simulink model "test"  (R2024a)
settings: Solver=ode1  StartTime=0.0  StopTime=4  FixedStep=0.0001  RelTol=1e-3  EnableMultiTasking=on
values from neighbouring files (symbols this model uses):
  kp = x(1)    [flc_error_ffunc.m]    (also in pi_regulator_ga_pso.m = wartosci_obliczone(1))
  ti = x(2)    [flc_error_ffunc.m]    (also in pi_regulator_ga_pso.m = wartosci_obliczone(2))
settings Model: Creator=poluser  LastModifiedBy=Hiver
settings DataIOCC: SaveOutput=off  SignalLogging=off  DSMLogging=off  SaveTime=off  ReturnWorkspaceOutputs=off
settings OptimizationCC: ReuseModelBlockBuffer=off
settings RTWCC: GPUComputeCapability=3.5

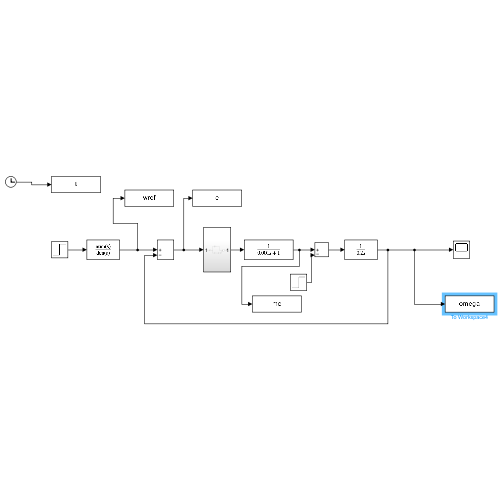
[thumbnail: Simulink's stored preview of the top-level diagram]
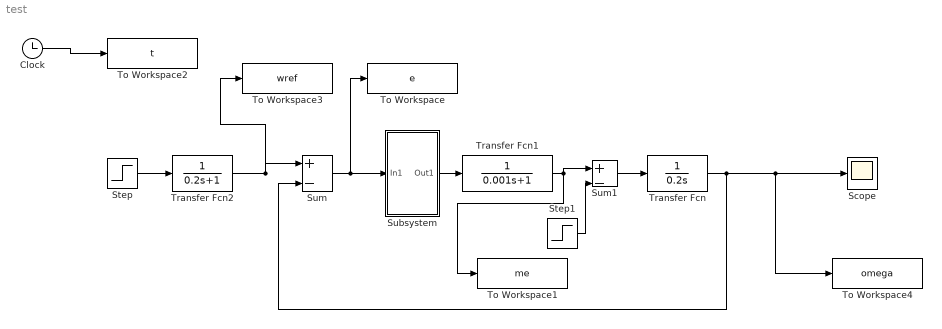
== system test ==
  Clock : Clock
  Scope : Scope
  Step : Step  Time=0.1  After=0.25  SampleTime=0
  Step1 : Step  SampleTime=0
  Subsystem : Subsystem
  Sum : Sum  Inputs=|+-
  Sum1 : Sum  Inputs=|+-
  To Workspace : ToWorkspace  VariableName=e  SampleTime=-1
  To Workspace1 : ToWorkspace  VariableName=me  SampleTime=-1
  To Workspace2 : ToWorkspace  VariableName=t  SampleTime=-1
  To Workspace3 : ToWorkspace  VariableName=wref  SampleTime=-1
  To Workspace4 : ToWorkspace  VariableName=omega  SampleTime=-1
  Transfer Fcn : TransferFcn  Denominator=[0.2 0]
  Transfer Fcn1 : TransferFcn  Denominator=[0.001 1]
  Transfer Fcn2 : TransferFcn  Denominator=[0.2 1]
  wires:
  Step/1 -> Transfer Fcn2/1
  Sum/1 -> Subsystem/1(In1), To Workspace/1
  Subsystem/1(Out1) -> Transfer Fcn1/1
  Transfer Fcn1/1 -> To Workspace1/1, Sum1/1
  Sum1/1 -> Transfer Fcn/1
  Transfer Fcn/1 -> Sum/2, To Workspace4/1, Scope/1
  Step1/1 -> Sum1/2
  Clock/1 -> To Workspace2/1
  Transfer Fcn2/1 -> To Workspace3/1, Sum/1

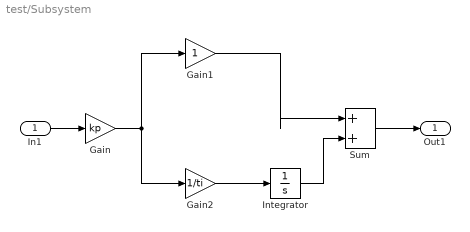
== system test/Subsystem ==
  In1 : Inport
  Gain : Gain  Gain=kp
  Gain1 : Gain
  Gain2 : Gain  Gain=1/ti
  Integrator : Integrator
  Sum : Sum  Inputs=|++
  Out1 : Outport
  wires:
  In1/1 -> Gain/1
  Gain/1 -> Gain2/1, Gain1/1
  Gain2/1 -> Integrator/1
  Integrator/1 -> Sum/2
  Gain1/1 -> Sum/1
  Sum/1 -> Out1/1
